simulink model "simulering_ROV_SM_controller"  (R2020a)
settings: Solver=ode45  StartTime=0.0  StopTime=t_sim  RelTol=1e-3
values from neighbouring files (symbols this model uses):
  B = [b11 b12 b13 b14 b15 b16 ... (first row only)    [constants.m]    (also in constants_dp_model.m; constants_model_coriolis.m; constants_process_model.m)
  B_psinv = B'/(B*B')    [constants_dp_model.m]    (also in constants_model_coriolis.m)
  d_11 = 250    [constants.m]    (also in constants_dp_model.m; constants_model_coriolis.m; constants_process_model.m)
  d_22 = 200    [constants.m]    (also in constants_dp_model.m; constants_model_coriolis.m; constants_process_model.m)
  d_33 = 175    [constants.m]    (also in constants_dp_model.m; constants_model_coriolis.m; constants_process_model.m)
  d_44 = 20    [constants.m]    (also in constants_dp_model.m = 15; constants_model_coriolis.m = 15; constants_process_model.m)
  g_z = 9.81    [run_simulation_FL_controller.m]    (also in run_simulation_PID_controller.m = 0.91; run_simulation_SM_controller.m = 0.91; run_simulation_STA_controller.m = 0.91; run_simulation_dp_model.m)
  gamma_r = 0.1    [run_simulation_FL_controller.m]    (also in run_simulation_PID_controller.m; run_simulation_SM_controller.m; run_simulation_STA_controller.m; run_simulation_feedback_linearizing.m)
  gamma_u = 0.1    [run_simulation_FL_controller.m]    (also in run_simulation_PID_controller.m; run_simulation_SM_controller.m; run_simulation_STA_controller.m; run_simulation_feedback_linearizing.m)
  gamma_v = 0.1    [run_simulation_FL_controller.m]    (also in run_simulation_PID_controller.m; run_simulation_SM_controller.m; run_simulation_STA_controller.m; run_simulation_feedback_linearizing.m)
  k_p_psi = wn_psi^2-lambda*k_p_r    [run_simulation_FL_controller.m]    (also in run_simulation_PID_controller.m = wn_psi^2*m_44; run_simulation_dp_model.m = wn_psi^2*m_44; run_simulation_feedback_linearizing.m = tau_r_max/deg2rad(45); run_simulation_feedback_linearizing_second_try.m = wn_psi^2*m_44)
  k_p_u = m_11*pole_u-d_11    [run_simulation_FL_controller.m]    (also in run_simulation_PID_controller.m = 10; run_simulation_dp_model.m = 3; run_simulation_feedback_linearizing.m = tau_u_max/100; run_simulation_feedback_linearizing_second_try.m = 1)
  k_p_v = m_22*pole_v-d_22    [run_simulation_FL_controller.m]    (also in run_simulation_PID_controller.m = 10; run_simulation_dp_model.m = 3; run_simulation_feedback_linearizing.m = tau_v_max/100; run_simulation_feedback_linearizing_second_try.m = 1)
  k_p_z = wn_heave^2*m_33    [run_simulation_PID_controller.m]    (also in tuning_FL_controller.m; tuning_PID_controller.m; tuning_dp_model.m)
  k_s_psi = 50    [run_simulation_SM_controller.m]    (also in tuning_SM_controller.m)
  k_s_u = 500    [run_simulation_SM_controller.m]    (also in tuning_SM_controller.m)
  k_s_v = 400    [run_simulation_SM_controller.m]    (also in tuning_SM_controller.m)
  k_s_z = 10    [run_simulation_SM_controller.m]    (also in tuning_SM_controller.m)
  lambda = d_44    [run_simulation_FL_controller.m]    (also in run_simulation_PID_controller.m = 1; run_simulation_SM_controller.m = 1; run_simulation_STA_controller.m = 1; run_simulation_feedback_linearizing.m = 1)
  lambda_psi = 1    [run_simulation_SM_controller.m]    (also in run_simulation_STA_controller.m = 0.5; tuning_SM_controller.m; tuning_STA_controller.m = 0.5)
  lambda_u = 0.5    [run_simulation_SM_controller.m]    (also in run_simulation_STA_controller.m = 10; tuning_SM_controller.m; tuning_STA_controller.m = 10)
  lambda_v = 0.5    [run_simulation_SM_controller.m]    (also in run_simulation_STA_controller.m = 10; tuning_SM_controller.m; tuning_STA_controller.m = 10)
  lambda_z = 3    [run_simulation_SM_controller.m]    (also in tuning_SM_controller.m)
  m_11 = m_RB11+m_A11    (= 144)    [constants.m]    (also in constants_dp_model.m; constants_model_coriolis.m; constants_process_model.m)
  m_22 = m_RB22+m_A22    (= 162)    [constants.m]    (also in constants_dp_model.m; constants_model_coriolis.m; constants_process_model.m)
  m_44 = m_RB44+m_A44    (= 21)    [constants.m]    (also in constants_dp_model.m = 18.2; constants_model_coriolis.m = 18.2; constants_process_model.m)
  m_A11 = 54    [constants.m]    (also in constants_dp_model.m; constants_model_coriolis.m; constants_process_model.m)
  m_A22 = 72    [constants.m]    (also in constants_dp_model.m; constants_model_coriolis.m; constants_process_model.m)
  m_A33 = 360    [constants.m]    (also in constants_dp_model.m; constants_model_coriolis.m; constants_process_model.m)
  m_A44 = 11    [constants.m]    (also in constants_dp_model.m = 5.2; constants_model_coriolis.m = 5.2; constants_process_model.m)
  m_RB11 = 90    [constants.m]    (also in constants_dp_model.m; constants_model_coriolis.m; constants_process_model.m)
  m_RB22 = 90    [constants.m]    (also in constants_dp_model.m; constants_model_coriolis.m; constants_process_model.m)
  m_RB33 = 90    [constants.m]    (also in constants_dp_model.m; constants_model_coriolis.m; constants_process_model.m)
  m_RB44 = 10    [constants.m]    (also in constants_dp_model.m = 13; constants_model_coriolis.m = 13; constants_process_model.m)
  phi_psi = 0.5    [run_simulation_SM_controller.m]    (also in tuning_SM_controller.m)
  phi_u = 1    [run_simulation_SM_controller.m]    (also in tuning_SM_controller.m)
  phi_v = 1    [run_simulation_SM_controller.m]    (also in tuning_SM_controller.m)
  phi_z = 0.5    [run_simulation_SM_controller.m]    (also in tuning_SM_controller.m)
  psi0 = deg2rad(psi0)    [constants.m]    (also in constants_dp_model.m; constants_model_coriolis.m; constants_process_model.m)
  r0 = 0    [constants.m]    (also in constants_dp_model.m; constants_model_coriolis.m; constants_process_model.m)
  u0 = 0    [constants.m]    (also in constants_dp_model.m; constants_model_coriolis.m; constants_process_model.m)
  v0 = 0    [constants.m]    (also in constants_dp_model.m; constants_model_coriolis.m; constants_process_model.m)
  V_x = 1    [constants.m]    (also in constants_process_model.m; run_simulation_FL_controller.m = 0.25; run_simulation_PID_controller.m = 0.25; run_simulation_dp_model.m = 0.25)
  V_y = 0    [constants.m]    (also in constants_process_model.m; run_simulation_FL_controller.m = -0.6; run_simulation_PID_controller.m = -0.6; run_simulation_dp_model.m = -0.6)
  w0 = 0    [constants.m]    (also in constants_dp_model.m; constants_model_coriolis.m; constants_process_model.m)
  x0 = -2*50    (= -100)    [constants.m]    (also in constants_dp_model.m = 0; constants_model_coriolis.m = 0; constants_process_model.m = 0)
  y0 = 0    [constants.m]    (also in constants_dp_model.m; constants_model_coriolis.m; constants_process_model.m)
  z0 = 0    [constants.m]    (also in constants_dp_model.m; constants_model_coriolis.m; constants_process_model.m)
settings Model: Creator=kenng  LastModifiedBy=kenng

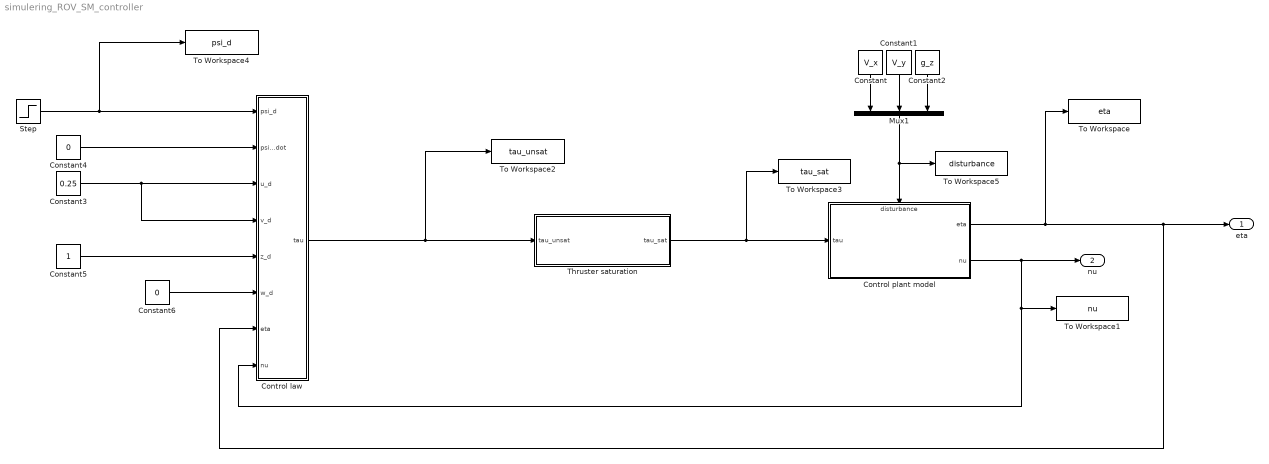
== system simulering_ROV_SM_controller ==
  Constant : Constant  Value=V_x
  Constant1 : Constant  Value=V_y
  Constant2 : Constant  Value=g_z
  Constant3 : Constant  Value=0.25
  Constant4 : Constant  Value=0
  Constant5 : Constant
  Constant6 : Constant  Value=0
  Control law : Subsystem
  Control plant model : Subsystem
      settings: PortSchema="{\"entries\":[{\"content\":{\"sides\":[{\"content\":{\"connectorIds\":[\"In1\"]},\"type\":\"ConnectorPlacement.EquallySpacedRectSide\",\"uuid\":\"e717a587-3200-458e-ba24-dd41565550b9\"},{\"content\":{\"connectorIds\":[\"Out1\",\"Out2\"],\"side\":\"RIGHT\"},\"type\":\"ConnectorPlacement.EquallySpacedRectSide\",\"uuid\":\"302c9cc9-c34e-45c2-bf93-40982187bd66\"},{\"content\":{\"connectorIds\":[\"In2\"],\"side\":\"TOP\"},\"type\":\"ConnectorPlacement.EquallySpacedRectSide\",\"uuid\":\"4b1c13ad-6fa1-447d-8a08-ad292496a8ea\"}]},\"type\":\"ConnectorPlacement.EquallySpacedConnector\",\"uuid\":\"78ff5622-69b9-4402-ac71-5e2cc2861626\"}],\"packageUris\":[\"http://schema.mathworks.com/mf0/Connector/19700101\"],\"version\":\"1.0\"}"
  Mux1 : Mux  Inputs=3
  Step : Step  Time=1000  Before=deg2rad(45)  After=deg2rad(90)  SampleTime=0
  Thruster saturation : Subsystem
  To Workspace : ToWorkspace  VariableName=eta  SaveFormat=Structure With Time  SampleTime=-1
  To Workspace1 : ToWorkspace  VariableName=nu  SaveFormat=Structure With Time  SampleTime=-1
  To Workspace2 : ToWorkspace  VariableName=tau_unsat  SaveFormat=Structure With Time  SampleTime=-1
  To Workspace3 : ToWorkspace  VariableName=tau_sat  SaveFormat=Structure With Time  SampleTime=-1
  To Workspace4 : ToWorkspace  VariableName=psi_d  SaveFormat=Structure With Time  SampleTime=-1
  To Workspace5 : ToWorkspace  VariableName=disturbance  SaveFormat=Structure With Time  SampleTime=-1
  eta : Outport
  nu : Outport  Port=2
  wires:
  Control plant model/1(eta) -> To Workspace/1, Control law/7(eta), eta/1
  Control plant model/2(nu) -> nu/1, To Workspace1/1, Control law/8(nu)
  Mux1/1 -> To Workspace5/1, Control plant model/2(disturbance)
  Control law/1(tau) -> Thruster saturation/1(tau_unsat), To Workspace2/1
  Step/1 -> To Workspace4/1, Control law/1(psi_d)
  Constant3/1 -> Control law/4(v_d), Control law/3(u_d)
  Constant/1 -> Mux1/1
  Constant1/1 -> Mux1/2
  Constant2/1 -> Mux1/3
  Constant5/1 -> Control law/5(z_d)
  Thruster saturation/1(tau_sat) -> To Workspace3/1, Control plant model/1(tau)
  Constant4/1 -> Control law/2(psi_d_dot)
  Constant6/1 -> Control law/6(w_d)

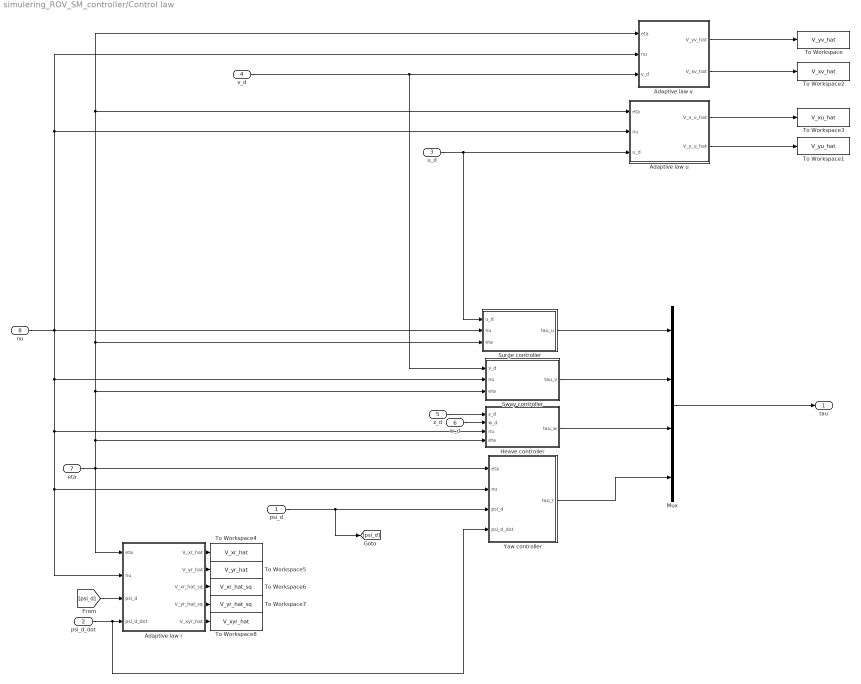
== system simulering_ROV_SM_controller/Control law ==
  psi_d : Inport
  psi_d_dot : Inport  Port=2
  u_d : Inport  Port=3
  v_d : Inport  Port=4
  z_d : Inport  Port=5
  w_d : Inport  Port=6
  eta : Inport  Port=7
  nu : Inport  Port=8
  Adaptive law r : Subsystem
  Adaptive law u : Subsystem
  Adaptive law v : Subsystem
  Heave controller : Subsystem
  Mux : Mux
  Surge controller : Subsystem
  Sway controller : Subsystem
  To Workspace : ToWorkspace  VariableName=V_yv_hat  SaveFormat=Structure With Time  SampleTime=-1
  To Workspace1 : ToWorkspace  VariableName=V_yu_hat  SaveFormat=Structure With Time  SampleTime=-1
  To Workspace2 : ToWorkspace  VariableName=V_xv_hat  SaveFormat=Structure With Time  SampleTime=-1
  To Workspace3 : ToWorkspace  VariableName=V_xu_hat  SaveFormat=Structure With Time  SampleTime=-1
  To Workspace4 : ToWorkspace  VariableName=V_xr_hat  SaveFormat=Structure With Time  SampleTime=-1
  To Workspace5 : ToWorkspace  VariableName=V_yr_hat  SaveFormat=Structure With Time  SampleTime=-1
  To Workspace6 : ToWorkspace  VariableName=V_xr_hat_sq  SaveFormat=Structure With Time  SampleTime=-1
  To Workspace7 : ToWorkspace  VariableName=V_yr_hat_sq  SaveFormat=Structure With Time  SampleTime=-1
  To Workspace8 : ToWorkspace  VariableName=V_xyr_hat  SaveFormat=Structure With Time  SampleTime=-1
  Yaw controller : Subsystem
  tau : Outport
  wires:
  Heave controller/1(tau_w) -> Mux/3
  Mux/1 -> tau/1
  u_d/1 -> Surge controller/1(u_d), Adaptive law u/3(u_d)
  v_d/1 -> Adaptive law v/3(v_d), Sway controller/1(v_d)
  z_d/1 -> Heave controller/1(z_d)
  Adaptive law u/2(V_y_u_hat) -> To Workspace1/1
  Adaptive law u/1(V_x_u_hat) -> To Workspace3/1
  Adaptive law v/1(V_yv_hat) -> To Workspace/1
  Adaptive law v/2(V_xv_hat) -> To Workspace2/1
  Adaptive law r/1(V_xr_hat) -> To Workspace4/1
  Adaptive law r/2(V_yr_hat) -> To Workspace5/1
  Adaptive law r/3(V_xr_hat_sq) -> To Workspace6/1
  Adaptive law r/4(V_yr_hat_sq) -> To Workspace7/1
  Adaptive law r/5(V_xyr_hat) -> To Workspace8/1
  [psi_d] -> Adaptive law r/3(psi_d)
  psi_d_dot/1 -> Yaw controller/4(psi_d_dot), Adaptive law r/4(psi_d_dot)
  eta/1 -> Adaptive law u/1(eta), Adaptive law v/1(eta), Surge controller/3(eta), Sway controller/3(eta), Heave controller/4(eta), Adaptive law r/1(eta), Yaw controller/1(eta)
  nu/1 -> Adaptive law r/2(nu), Yaw controller/2(nu), Heave controller/3(nu), Sway controller/2(nu), Adaptive law u/2(nu), Adaptive law v/2(nu), Surge controller/2(nu)
  psi_d/1 -> Yaw controller/3(psi_d), [psi_d]
  Yaw controller/1(tau_r) -> Mux/4
  Surge controller/1(tau_u) -> Mux/1
  Sway controller/1(tau_v) -> Mux/2
  w_d/1 -> Heave controller/2(w_d)

== system simulering_ROV_SM_controller/Control plant model ==
  note: tau: 4x1 vector = [surge sway heave yaw]^T
  note: Disturbance: 3x1 vector = [Vx Vy gz]^t
  tau : Inport
  disturbance : Inport  Port=2
  Demux : Demux
  Kinematics : Subsystem
  Kinetics : Subsystem
  Terminator : Terminator
  Terminator1 : Terminator
  Terminator2 : Terminator
  eta : Outport
  nu : Outport  Port=2
  wires:
  tau/1 -> Kinetics/2(tau)
  Kinetics/1(nu) -> nu/1, Kinematics/1(nu)
  Demux/4 -> Kinetics/3(psi)
  Demux/2 -> Terminator1/1
  Kinematics/1(eta) -> eta/1, Demux/1
  Demux/1 -> Terminator/1
  Demux/3 -> Terminator2/1
  disturbance/1 -> Kinetics/1(disturbance)

== system simulering_ROV_SM_controller/Thruster saturation ==
  tau_unsat : Inport
  Constant : Constant  Value=B_psinv
  Constant1 : Constant  Value=B
  Demux : Demux  Outputs=6
  Matrix Multiply : Product  Multiplication=Matrix(*)
  Matrix Multiply1 : Product  Multiplication=Matrix(*)
  Mux : Mux  Inputs=6
  Saturation{,1..5} (6 alike) : Saturate  UpperLimit=120  LowerLimit=-120
  tau_sat : Outport
  wires:
  tau_unsat/1 -> Matrix Multiply/2
  Constant/1 -> Matrix Multiply/1
  Matrix Multiply/1 -> Demux/1
  Demux/2 -> Saturation1/1
  Demux/1 -> Saturation/1
  Demux/3 -> Saturation2/1
  Demux/4 -> Saturation3/1
  Demux/5 -> Saturation4/1
  Demux/6 -> Saturation5/1
  Saturation/1 -> Mux/1
  Saturation1/1 -> Mux/2
  Saturation2/1 -> Mux/3
  Saturation3/1 -> Mux/4
  Saturation4/1 -> Mux/5
  Saturation5/1 -> Mux/6
  Mux/1 -> Matrix Multiply1/2
  Constant1/1 -> Matrix Multiply1/1
  Matrix Multiply1/1 -> tau_sat/1

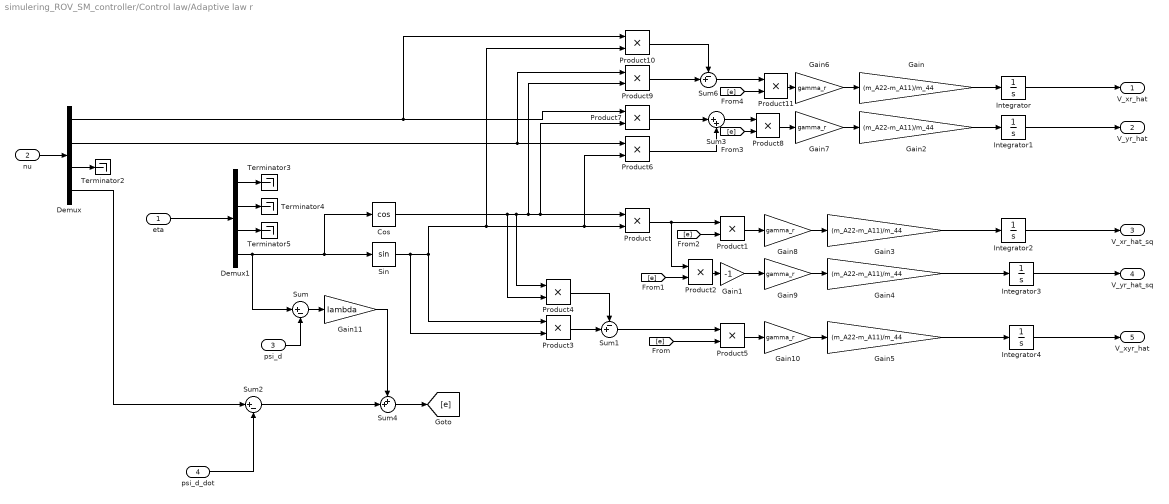
== system simulering_ROV_SM_controller/Control law/Adaptive law r ==
  eta : Inport
  nu : Inport  Port=2
  psi_d : Inport  Port=3
  psi_d_dot : Inport  Port=4
  Cos : Trigonometry  Operator=cos
  Demux : Demux
  Demux1 : Demux
  Gain{,2..5} (5 alike) : Gain  Gain=(m_A22-m_A11)/m_44
  Gain1 : Gain  Gain=-1
  Gain{6..10} (5 alike) : Gain  Gain=gamma_r
  Gain11 : Gain  Gain=lambda
  Integrator{,1..4} (5 alike) : Integrator
  Product{,1..11} (12 alike) : Product
  Sin : Trigonometry
  Sum : Sum  Inputs=|+-
  Sum1 : Sum  Inputs=-+|
  Sum2 : Sum  Inputs=|+-
  Sum3 : Sum  Inputs=|++
  Sum4 : Sum  Inputs=++|
  Sum6 : Sum  Inputs=-+|
  Terminator{2..5} (4 alike) : Terminator
  V_xr_hat : Outport
  V_yr_hat : Outport  Port=2
  V_xr_hat_sq : Outport  Port=3
  V_yr_hat_sq : Outport  Port=4
  V_xyr_hat : Outport  Port=5
  wires:
  [e] -> Product11/2
  [e] -> Product8/2
  nu/1 -> Demux/1
  Demux/1 -> Product10/1, Product7/1
  Demux/2 -> Product9/1, Product6/1
  Demux/3 -> Terminator2/1
  Demux1/2 -> Terminator4/1
  eta/1 -> Demux1/1
  Demux1/1 -> Terminator3/1
  Demux1/3 -> Terminator5/1
  Demux1/4 -> Cos/1, Sin/1, Sum/1
  Demux/4 -> Sum2/1
  Sin/1 -> Product3/2, Product3/1, Product10/2, Product6/2, Product/2
  Cos/1 -> Product4/2, Product4/1, Product9/2, Product7/2, Product/1
  [e] -> Product1/2
  Product1/1 -> Gain8/1
  Product2/1 -> Gain1/1
  [e] -> Product2/2
  Product/1 -> Product2/1, Product1/1
  Product3/1 -> Sum1/2
  Product4/1 -> Sum1/1
  Sum1/1 -> Product5/1
  [e] -> Product5/2
  Product7/1 -> Sum3/1
  Product6/1 -> Sum3/2
  Sum3/1 -> Product8/1
  Product9/1 -> Sum6/2
  Product10/1 -> Sum6/1
  Sum6/1 -> Product11/1
  Gain1/1 -> Gain9/1
  Product11/1 -> Gain6/1
  Product8/1 -> Gain7/1
  Product5/1 -> Gain10/1
  Gain/1 -> Integrator/1
  Gain2/1 -> Integrator1/1
  Gain3/1 -> Integrator2/1
  Gain4/1 -> Integrator3/1
  Gain5/1 -> Integrator4/1
  Integrator4/1 -> V_xyr_hat/1
  Integrator3/1 -> V_yr_hat_sq/1
  Integrator2/1 -> V_xr_hat_sq/1
  Integrator1/1 -> V_yr_hat/1
  Integrator/1 -> V_xr_hat/1
  Gain6/1 -> Gain/1
  Gain7/1 -> Gain2/1
  Gain8/1 -> Gain3/1
  Gain9/1 -> Gain4/1
  Gain10/1 -> Gain5/1
  psi_d_dot/1 -> Sum2/2
  psi_d/1 -> Sum/2
  Sum/1 -> Gain11/1
  Sum2/1 -> Sum4/2
  Gain11/1 -> Sum4/1
  Sum4/1 -> [e]

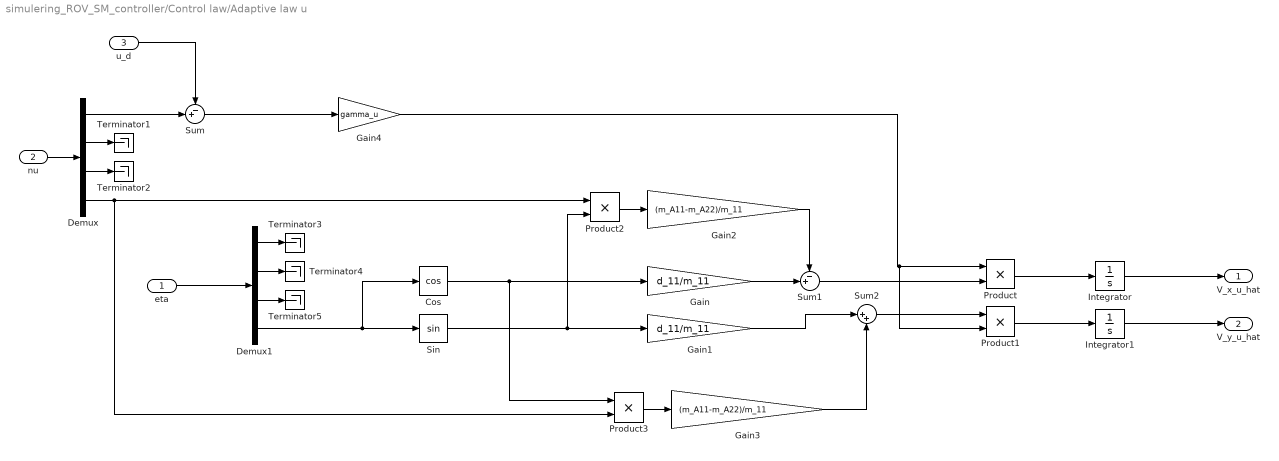
== system simulering_ROV_SM_controller/Control law/Adaptive law u ==
  eta : Inport
  nu : Inport  Port=2
  u_d : Inport  Port=3
  Cos : Trigonometry  Operator=cos
  Demux : Demux
  Demux1 : Demux
  Gain : Gain  Gain=d_11/m_11
  Gain1 : Gain  Gain=d_11/m_11
  Gain2 : Gain  Gain=(m_A11-m_A22)/m_11
  Gain3 : Gain  Gain=(m_A11-m_A22)/m_11
  Gain4 : Gain  Gain=gamma_u
  Integrator : Integrator
  Integrator1 : Integrator
  Product{,1..3} (4 alike) : Product
  Sin : Trigonometry
  Sum : Sum  Inputs=-+|
  Sum1 : Sum  Inputs=-+|
  Sum2 : Sum  Inputs=|++
  Terminator{1..5} (5 alike) : Terminator
  V_x_u_hat : Outport
  V_y_u_hat : Outport  Port=2
  wires:
  Sin/1 -> Product2/2, Gain1/1
  Product/1 -> Integrator/1
  Product1/1 -> Integrator1/1
  Gain4/1 -> Product1/2, Product/1
  Integrator/1 -> V_x_u_hat/1
  Gain/1 -> Sum1/2
  Sum1/1 -> Product/2
  Gain2/1 -> Sum1/1
  nu/1 -> Demux/1
  Product2/1 -> Gain2/1
  Sum2/1 -> Product1/1
  Gain1/1 -> Sum2/1
  Product3/1 -> Gain3/1
  Cos/1 -> Product3/1, Gain/1
  Gain3/1 -> Sum2/2
  Demux/4 -> Product2/1, Product3/2
  Demux/1 -> Sum/2
  Demux/2 -> Terminator1/1
  Demux/3 -> Terminator2/1
  Demux1/2 -> Terminator4/1
  eta/1 -> Demux1/1
  Demux1/1 -> Terminator3/1
  Demux1/3 -> Terminator5/1
  Demux1/4 -> Cos/1, Sin/1
  u_d/1 -> Sum/1
  Sum/1 -> Gain4/1
  Integrator1/1 -> V_y_u_hat/1

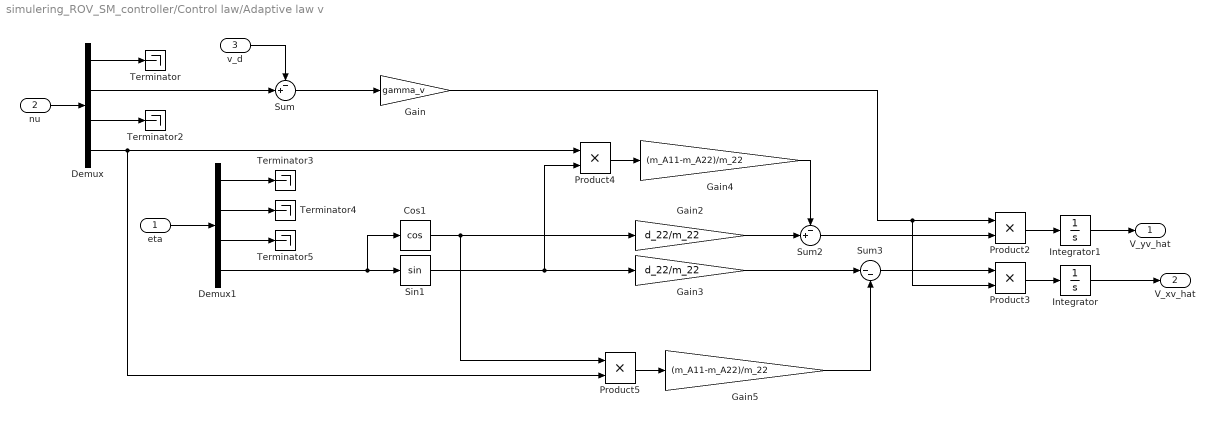
== system simulering_ROV_SM_controller/Control law/Adaptive law v ==
  eta : Inport
  nu : Inport  Port=2
  v_d : Inport  Port=3
  Cos1 : Trigonometry  Operator=cos
  Demux : Demux
  Demux1 : Demux
  Gain : Gain  Gain=gamma_v
  Gain2 : Gain  Gain=d_22/m_22
  Gain3 : Gain  Gain=d_22/m_22
  Gain4 : Gain  Gain=(m_A11-m_A22)/m_22
  Gain5 : Gain  Gain=(m_A11-m_A22)/m_22
  Integrator : Integrator
  Integrator1 : Integrator
  Product{2..5} (4 alike) : Product
  Sin1 : Trigonometry
  Sum : Sum  Inputs=-+|
  Sum2 : Sum  Inputs=-+|
  Sum3 : Sum  Inputs=|--
  Terminator{,2..5} (5 alike) : Terminator
  V_yv_hat : Outport
  V_xv_hat : Outport  Port=2
  wires:
  Gain4/1 -> Sum2/1
  Product5/1 -> Gain5/1
  Gain2/1 -> Sum2/2
  Demux/3 -> Terminator2/1
  Product4/1 -> Gain4/1
  nu/1 -> Demux/1
  Gain5/1 -> Sum3/2
  Sum2/1 -> Product2/2
  Integrator1/1 -> V_yv_hat/1
  Gain/1 -> Product3/2, Product2/1
  Product2/1 -> Integrator1/1
  Sum3/1 -> Product3/1
  Demux/2 -> Sum/2
  Demux/1 -> Terminator/1
  Gain3/1 -> Sum3/1
  Demux/4 -> Product4/1, Product5/2
  Cos1/1 -> Product5/1, Gain2/1
  Sin1/1 -> Product4/2, Gain3/1
  Demux1/1 -> Terminator3/1
  Demux1/2 -> Terminator4/1
  eta/1 -> Demux1/1
  Demux1/3 -> Terminator5/1
  Demux1/4 -> Cos1/1, Sin1/1
  Product3/1 -> Integrator/1
  Integrator/1 -> V_xv_hat/1
  v_d/1 -> Sum/1
  Sum/1 -> Gain/1

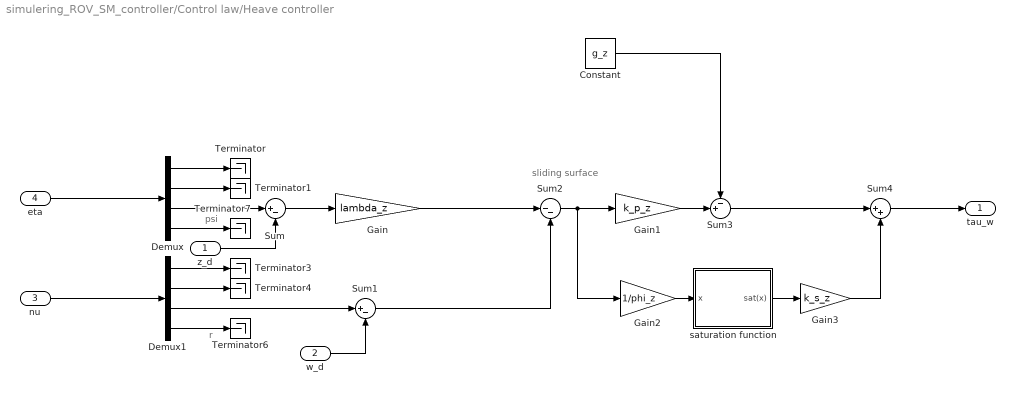
== system simulering_ROV_SM_controller/Control law/Heave controller ==
  note: sliding surface
  note: r
  note: psi
  z_d : Inport
  w_d : Inport  Port=2
  nu : Inport  Port=3
  eta : Inport  Port=4
  Constant : Constant  Value=g_z
  Demux : Demux
  Demux1 : Demux
  Gain : Gain  Gain=lambda_z
  Gain1 : Gain  Gain=k_p_z
  Gain2 : Gain  Gain=1/phi_z
  Gain3 : Gain  Gain=k_s_z
  Sum : Sum  Inputs=|+-
  Sum1 : Sum  Inputs=|+-
  Sum2 : Sum  Inputs=|--
  Sum3 : Sum  Inputs=-+|
  Sum4 : Sum  Inputs=|++
  Terminator{,1,3..4,6..7} (6 alike) : Terminator
  saturation function : Subsystem
  tau_w : Outport
  wires:
  Demux1/2 -> Terminator4/1
  Demux/1 -> Terminator/1
  eta/1 -> Demux/1
  Demux/2 -> Terminator1/1
  Demux1/1 -> Terminator3/1
  Demux/3 -> Sum/1
  nu/1 -> Demux1/1
  Demux1/4 -> Terminator6/1
  Demux/4 -> Terminator7/1
  z_d/1 -> Sum/2
  Sum/1 -> Gain/1
  Demux1/3 -> Sum1/1
  w_d/1 -> Sum1/2
  Gain/1 -> Sum2/1
  Sum1/1 -> Sum2/2
  Sum2/1 -> Gain2/1, Gain1/1
  Constant/1 -> Sum3/1
  Gain1/1 -> Sum3/2
  Gain2/1 -> saturation function/1(x)
  Sum3/1 -> Sum4/1
  saturation function/1(sat(x)) -> Gain3/1
  Gain3/1 -> Sum4/2
  Sum4/1 -> tau_w/1

== system simulering_ROV_SM_controller/Control law/Surge controller ==
  note: sliding surface
  note: r
  note: psi
  u_d : Inport
  nu : Inport  Port=2
  eta : Inport  Port=3
  Demux : Demux
  Demux1 : Demux
  Gain : Gain  Gain=lambda_u
  Gain1 : Gain  Gain=k_p_u
  Gain2 : Gain  Gain=1/phi_u
  Gain3 : Gain  Gain=k_s_u
  Integrator : Integrator
  Sum : Sum  Inputs=|+-
  Sum1 : Sum  Inputs=|--
  Sum2 : Sum  Inputs=|++
  Terminator{,1..2,4..7} (7 alike) : Terminator
  saturation function : Subsystem
  tau_u : Outport
  wires:
  Demux1/2 -> Terminator4/1
  eta/1 -> Demux/1
  Demux/2 -> Terminator1/1
  Demux1/1 -> Sum/1
  nu/1 -> Demux1/1
  Demux1/4 -> Terminator6/1
  Demux/4 -> Terminator7/1
  u_d/1 -> Sum/2
  Demux1/3 -> Terminator2/1
  Demux/3 -> Terminator/1
  Demux/1 -> Terminator5/1
  Sum/1 -> Integrator/1, Sum1/2
  Integrator/1 -> Gain/1
  Gain/1 -> Sum1/1
  Sum1/1 -> Gain2/1, Gain1/1
  Gain2/1 -> saturation function/1(x)
  saturation function/1(sat(x)) -> Gain3/1
  Gain1/1 -> Sum2/1
  Gain3/1 -> Sum2/2
  Sum2/1 -> tau_u/1

== system simulering_ROV_SM_controller/Control law/Sway controller ==
  note: sliding surface
  note: r
  note: psi
  v_d : Inport
  nu : Inport  Port=2
  eta : Inport  Port=3
  Demux : Demux
  Demux1 : Demux
  Gain : Gain  Gain=k_p_v
  Gain1 : Gain  Gain=lambda_v
  Gain2 : Gain  Gain=1/phi_v
  Gain3 : Gain  Gain=k_s_v
  Integrator : Integrator
  Sum : Sum  Inputs=|+-
  Sum1 : Sum  Inputs=|--
  Sum2 : Sum  Inputs=|++
  Terminator{,1..3,5..7} (7 alike) : Terminator
  saturation function : Subsystem
  tau_v : Outport
  wires:
  Demux1/2 -> Sum/1
  Demux/1 -> Terminator/1
  eta/1 -> Demux/1
  Demux1/1 -> Terminator3/1
  nu/1 -> Demux1/1
  Demux1/4 -> Terminator6/1
  Demux/4 -> Terminator7/1
  v_d/1 -> Sum/2
  Gain/1 -> Sum2/1
  Demux1/3 -> Terminator2/1
  Demux/3 -> Terminator1/1
  Demux/2 -> Terminator5/1
  Sum/1 -> Sum1/2, Integrator/1
  Integrator/1 -> Gain1/1
  Sum1/1 -> Gain2/1, Gain/1
  Gain2/1 -> saturation function/1(x)
  saturation function/1(sat(x)) -> Gain3/1
  Gain3/1 -> Sum2/2
  Sum2/1 -> tau_v/1
  Gain1/1 -> Sum1/1

== system simulering_ROV_SM_controller/Control law/Yaw controller ==
  note: sliding surface
  note: r
  note: psi
  eta : Inport
  nu : Inport  Port=2
  psi_d : Inport  Port=3
  psi_d_dot : Inport  Port=4
  Demux : Demux
  Demux1 : Demux
  Gain : Gain  Gain=lambda_psi
  Gain1 : Gain  Gain=1/phi_psi
  Gain2 : Gain  Gain=k_p_psi
  Gain3 : Gain  Gain=k_s_psi
  SSA : MATLAB Function  TreatAsAtomicUnit=on
  Sum : Sum  Inputs=|+-
  Sum1 : Sum  Inputs=|+-
  Sum2 : Sum  Inputs=|--
  Sum4 : Sum  Inputs=|++
  Terminator{,1..5} (6 alike) : Terminator
  saturation function : Subsystem
  tau_r : Outport
  wires:
  Demux/2 -> Terminator1/1
  Demux/1 -> Terminator/1
  Demux1/1 -> Terminator3/1
  Demux1/3 -> Terminator2/1
  Demux1/2 -> Terminator4/1
  eta/1 -> Demux/1
  nu/1 -> Demux1/1
  Demux/3 -> Terminator5/1
  Gain2/1 -> Sum4/1
  Sum4/1 -> tau_r/1
  psi_d/1 -> Sum/2
  Demux/4 -> Sum/1
  Demux1/4 -> Sum1/1
  psi_d_dot/1 -> Sum1/2
  Sum/1 -> SSA/1(u)
  Gain/1 -> Sum2/1
  Sum1/1 -> Sum2/2
  Sum2/1 -> Gain1/1, Gain2/1
  Gain1/1 -> saturation function/1(x)
  saturation function/1(sat(x)) -> Gain3/1
  Gain3/1 -> Sum4/2
  SSA/1(y) -> Gain/1

== system simulering_ROV_SM_controller/Control plant model/Kinematics ==
  nu : Inport
  Cos : Trigonometry  Operator=cos
  Demux : Demux
  Integrator : Integrator  InitialCondition=psi0
  Integrator1 : Integrator  InitialCondition=z0
  Integrator2 : Integrator  InitialCondition=x0
  Integrator3 : Integrator  InitialCondition=y0
  Mux : Mux
  Product{,1..3} (4 alike) : Product
  Sin : Trigonometry
  Sum : Sum  Inputs=|++
  Sum1 : Sum  Inputs=|+-
  eta : Outport
  wires:
  Sin/1 -> [sinpsi]
  Demux/3 -> Integrator1/1
  Demux/1 -> Product1/1, Product/1
  Demux/2 -> Product3/1, Product2/1
  [sinpsi] -> Product3/2
  [psi] -> Sin/1, Cos/1
  [cospsi] -> Product2/2
  Cos/1 -> [cospsi]
  Product1/1 -> Sum/1
  Integrator/1 -> Mux/4, [psi]
  [sinpsi] -> Product1/2
  Product/1 -> Sum1/1
  Sum1/1 -> Integrator2/1
  Demux/4 -> Integrator/1
  Sum/1 -> Integrator3/1
  [cospsi] -> Product/2
  nu/1 -> Demux/1
  Product2/1 -> Sum/2
  Product3/1 -> Sum1/2
  Integrator3/1 -> Mux/2
  Integrator1/1 -> Mux/3
  Integrator2/1 -> Mux/1
  Mux/1 -> eta/1

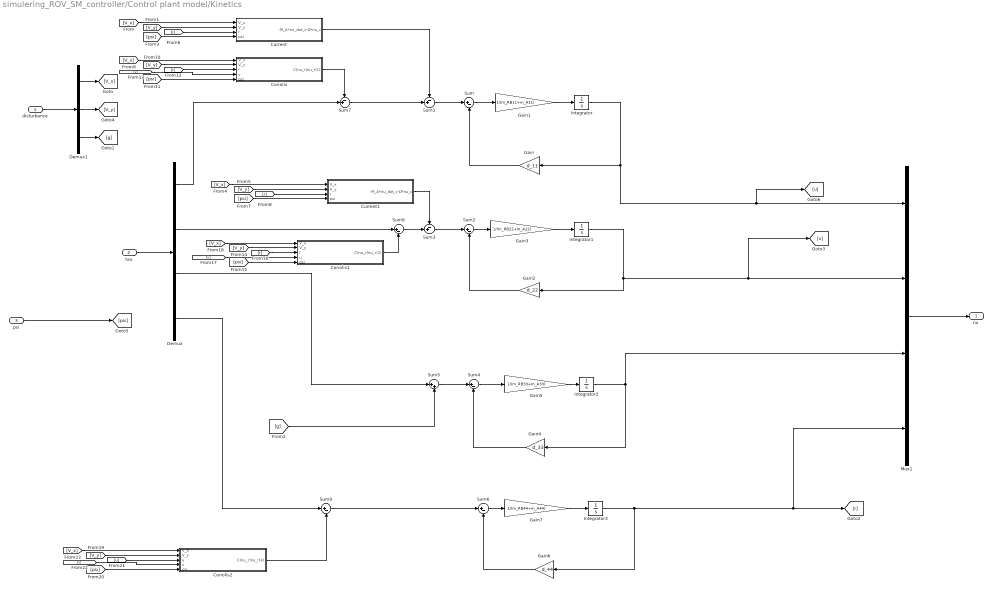
== system simulering_ROV_SM_controller/Control plant model/Kinetics ==
  disturbance : Inport
  tau : Inport  Port=2
  psi : Inport  Port=3
  Coriolis : Subsystem
  Coriolis1 : Subsystem
  Coriolis2 : Subsystem
  Current : Subsystem
  Current1 : Subsystem
  Demux : Demux
  Demux1 : Demux  Outputs=3
  Gain : Gain  Gain=d_11
  Gain1 : Gain  Gain=1/(m_RB11+m_A11)
  Gain2 : Gain  Gain=d_22
  Gain3 : Gain  Gain=1/(m_RB22+m_A22)
  Gain4 : Gain  Gain=d_33
  Gain5 : Gain  Gain=1/(m_RB33+m_A33)
  Gain6 : Gain  Gain=d_44
  Gain7 : Gain  Gain=1/(m_RB44+m_A44)
  Integrator : Integrator  InitialCondition=u0
  Integrator1 : Integrator  InitialCondition=v0
  Integrator2 : Integrator  InitialCondition=w0
  Integrator3 : Integrator  InitialCondition=r0
  Mux1 : Mux
  Sum{,2,4,6,8..9} (6 alike) : Sum  Inputs=|+-
  Sum1 : Sum  Inputs=-+|
  Sum3 : Sum  Inputs=-+|
  Sum5 : Sum  Inputs=|++
  Sum7 : Sum  Inputs=-+|
  nu : Outport
  wires:
  Demux1/1 -> [V_x]
  Gain1/1 -> Integrator/1
  Sum/1 -> Gain1/1
  tau/1 -> Demux/1
  Integrator1/1 -> Gain2/1, [v], Mux1/2
  Gain3/1 -> Integrator1/1
  Mux1/1 -> nu/1
  Integrator/1 -> [u], Mux1/1, Gain/1
  Integrator2/1 -> Gain4/1, Mux1/3
  Gain5/1 -> Integrator2/1
  Demux1/3 -> [g]
  Sum3/1 -> Sum2/1
  Sum4/1 -> Gain5/1
  Gain2/1 -> Sum2/2
  Sum2/1 -> Gain3/1
  Gain/1 -> Sum/2
  Gain4/1 -> Sum4/2
  Sum1/1 -> Sum/1
  Gain6/1 -> Sum6/2
  Demux1/2 -> [V_y]
  [r] -> Current/3(r)
  Integrator3/1 -> [r], Mux1/4, Gain6/1
  disturbance/1 -> Demux1/1
  Sum6/1 -> Gain7/1
  Gain7/1 -> Integrator3/1
  psi/1 -> [psi]
  Current/1(-M_A*nu_dot_c-D*nu_c) -> Sum1/1
  [V_y] -> Current/2(V_y)
  [V_x] -> Current/1(V_x)
  [psi] -> Current/4(psi)
  [r] -> Current1/3(r)
  [psi] -> Current1/4(psi)
  [V_x] -> Current1/1(V_x)
  [V_y] -> Current1/2(V_y)
  Current1/1(-M_A*nu_dot_c-D*nu_c) -> Sum3/1
  [g] -> Sum5/2
  Demux/3 -> Sum5/1
  Sum5/1 -> Sum4/1
  Coriolis/1(C(nu_r)nu_r(1)) -> Sum7/1
  Demux/1 -> Sum7/2
  Sum7/1 -> Sum1/2
  [V_x] -> Coriolis/1(V_x)
  [psi] -> Coriolis/5(psi)
  [r] -> Coriolis/3(r)
  [V_y] -> Coriolis/2(V_y)
  [v] -> Coriolis/4(v)
  [u] -> Coriolis1/4(u)
  Coriolis1/1(C(nu_r)nu_r(2)) -> Sum8/2
  [V_y] -> Coriolis1/2(V_y)
  [psi] -> Coriolis1/5(psi)
  [V_x] -> Coriolis1/1(V_x)
  [r] -> Coriolis1/3(r)
  Sum8/1 -> Sum3/2
  Demux/2 -> Sum8/1
  [v] -> Coriolis2/4(v)
  Coriolis2/1(C(nu_r)nu_r(4)) -> Sum9/2
  [V_y] -> Coriolis2/2(V_y)
  [psi] -> Coriolis2/5(psi)
  [V_x] -> Coriolis2/1(V_x)
  [u] -> Coriolis2/3(u)
  Sum9/1 -> Sum6/1
  Demux/4 -> Sum9/1

== system simulering_ROV_SM_controller/Control law/Heave controller/saturation function ==
  x : Inport
  Abs : Abs
  Sign : Signum
  Switch : Switch  Criteria=u2 > Threshold  Threshold=1
  sat(x) : Outport
  wires:
  x/1 -> Sign/1, Abs/1, Switch/3
  Abs/1 -> Switch/2
  Sign/1 -> Switch/1
  Switch/1 -> sat(x)/1

== system simulering_ROV_SM_controller/Control law/Surge controller/saturation function ==
  x : Inport
  Abs : Abs
  Sign : Signum
  Switch : Switch  Criteria=u2 > Threshold  Threshold=1
  sat(x) : Outport
  wires:
  x/1 -> Sign/1, Abs/1, Switch/3
  Abs/1 -> Switch/2
  Sign/1 -> Switch/1
  Switch/1 -> sat(x)/1

== system simulering_ROV_SM_controller/Control law/Sway controller/saturation function ==
  x : Inport
  Abs : Abs
  Sign : Signum
  Switch : Switch  Criteria=u2 > Threshold  Threshold=1
  sat(x) : Outport
  wires:
  x/1 -> Sign/1, Abs/1, Switch/3
  Abs/1 -> Switch/2
  Sign/1 -> Switch/1
  Switch/1 -> sat(x)/1

== system simulering_ROV_SM_controller/Control law/Yaw controller/saturation function ==
  x : Inport
  Abs : Abs
  Sign : Signum
  Switch : Switch  Criteria=u2 > Threshold  Threshold=1
  sat(x) : Outport
  wires:
  x/1 -> Sign/1, Abs/1, Switch/3
  Abs/1 -> Switch/2
  Sign/1 -> Switch/1
  Switch/1 -> sat(x)/1

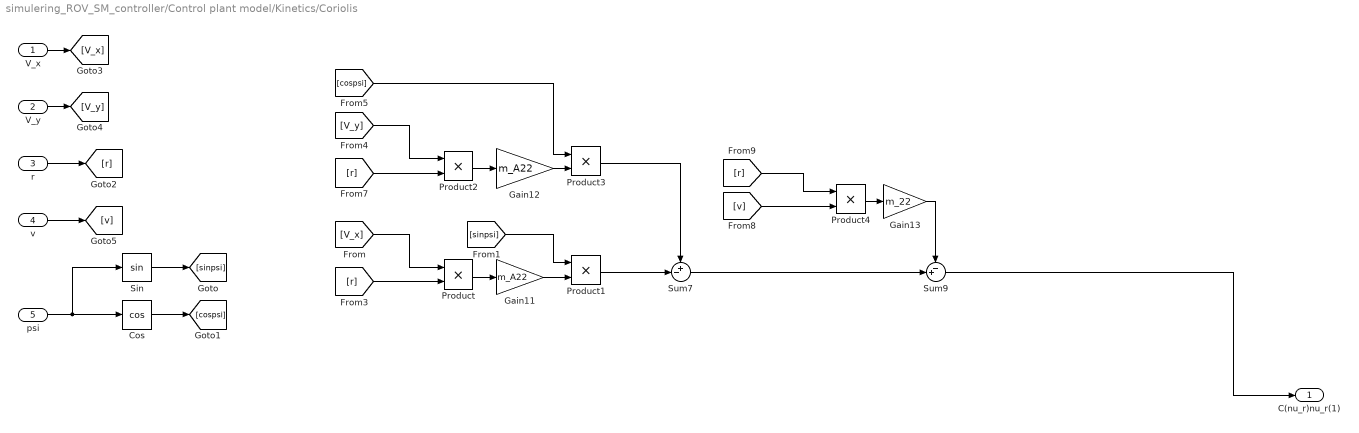
== system simulering_ROV_SM_controller/Control plant model/Kinetics/Coriolis ==
  V_x : Inport
  V_y : Inport  Port=2
  r : Inport  Port=3
  v : Inport  Port=4
  psi : Inport  Port=5
  Cos : Trigonometry  Operator=cos
  Gain11 : Gain  Gain=m_A22
  Gain12 : Gain  Gain=m_A22
  Gain13 : Gain  Gain=m_22
  Product{,1..4} (5 alike) : Product
  Sin : Trigonometry
  Sum7 : Sum  Inputs=+-|
  Sum9 : Sum  Inputs=-+|
  C(nu_r)nu_r(1) : Outport
  wires:
  Gain11/1 -> Product1/2
  Product2/1 -> Gain12/1
  [cospsi] -> Product3/1
  [r] -> Product2/2
  [v] -> Product4/2
  Product4/1 -> Gain13/1
  [V_x] -> Product/1
  Product3/1 -> Sum7/1
  Gain12/1 -> Product3/2
  Product/1 -> Gain11/1
  [V_y] -> Product2/1
  [r] -> Product/2
  Product1/1 -> Sum7/2
  [sinpsi] -> Product1/1
  Sum7/1 -> Sum9/2
  [r] -> Product4/1
  Sum9/1 -> C(nu_r)nu_r(1)/1
  psi/1 -> Sin/1, Cos/1
  Sin/1 -> [sinpsi]
  Cos/1 -> [cospsi]
  r/1 -> [r]
  V_x/1 -> [V_x]
  V_y/1 -> [V_y]
  v/1 -> [v]
  Gain13/1 -> Sum9/1

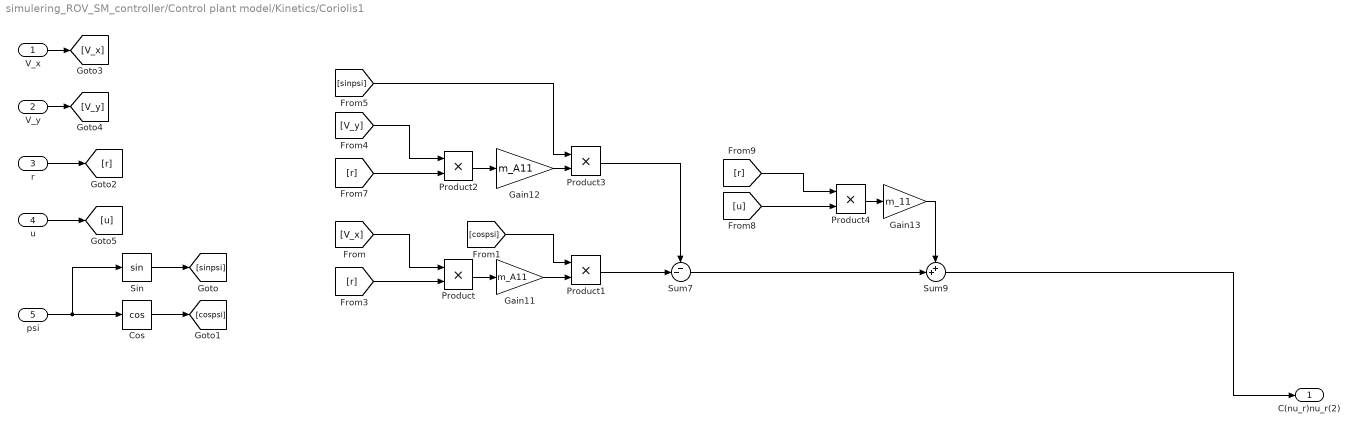
== system simulering_ROV_SM_controller/Control plant model/Kinetics/Coriolis1 ==
  V_x : Inport
  V_y : Inport  Port=2
  r : Inport  Port=3
  u : Inport  Port=4
  psi : Inport  Port=5
  Cos : Trigonometry  Operator=cos
  Gain11 : Gain  Gain=m_A11
  Gain12 : Gain  Gain=m_A11
  Gain13 : Gain  Gain=m_11
  Product{,1..4} (5 alike) : Product
  Sin : Trigonometry
  Sum7 : Sum  Inputs=--|
  Sum9 : Sum  Inputs=++|
  C(nu_r)nu_r(2) : Outport
  wires:
  Gain11/1 -> Product1/2
  Product2/1 -> Gain12/1
  [sinpsi] -> Product3/1
  [r] -> Product2/2
  [u] -> Product4/2
  Product4/1 -> Gain13/1
  [V_x] -> Product/1
  Product3/1 -> Sum7/1
  Gain12/1 -> Product3/2
  Product/1 -> Gain11/1
  [V_y] -> Product2/1
  [r] -> Product/2
  Product1/1 -> Sum7/2
  [cospsi] -> Product1/1
  Sum7/1 -> Sum9/2
  [r] -> Product4/1
  Sum9/1 -> C(nu_r)nu_r(2)/1
  psi/1 -> Sin/1, Cos/1
  Sin/1 -> [sinpsi]
  Cos/1 -> [cospsi]
  r/1 -> [r]
  V_x/1 -> [V_x]
  V_y/1 -> [V_y]
  u/1 -> [u]
  Gain13/1 -> Sum9/1

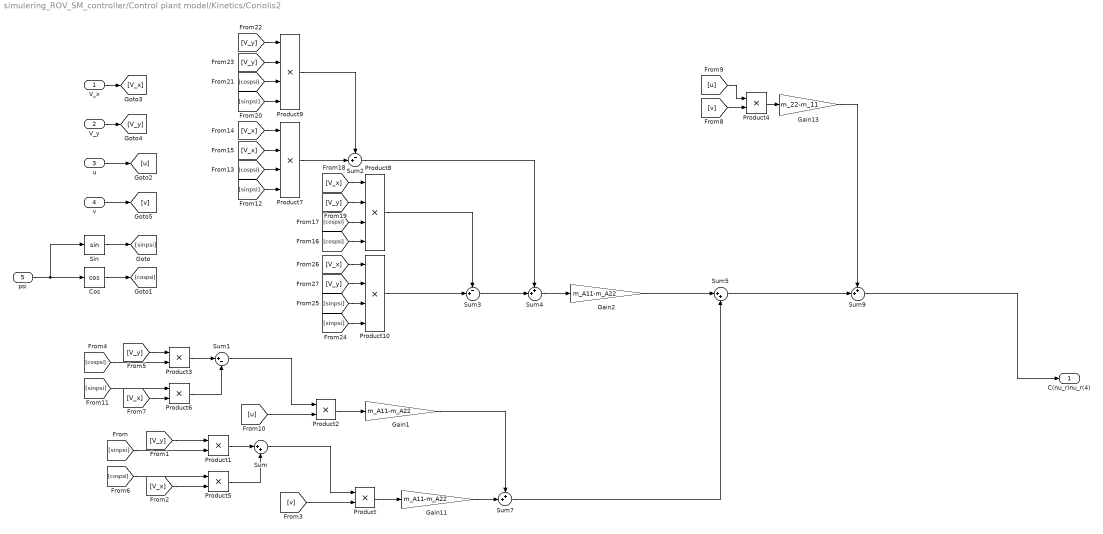
== system simulering_ROV_SM_controller/Control plant model/Kinetics/Coriolis2 ==
  V_x : Inport
  V_y : Inport  Port=2
  u : Inport  Port=3
  v : Inport  Port=4
  psi : Inport  Port=5
  Cos : Trigonometry  Operator=cos
  Gain1 : Gain  Gain=m_A11-m_A22
  Gain11 : Gain  Gain=m_A11-m_A22
  Gain13 : Gain  Gain=m_22-m_11
  Gain2 : Gain  Gain=m_A11-m_A22
  Product{,1..6} (7 alike) : Product
  Product{7..10} (4 alike) : Product  Inputs=4
  Sin : Trigonometry
  Sum : Sum  Inputs=|++
  Sum1 : Sum  Inputs=|+-
  Sum2 : Sum  Inputs=-+|
  Sum3 : Sum  Inputs=-+|
  Sum4 : Sum  Inputs=++|
  Sum5 : Sum  Inputs=|++
  Sum7 : Sum  Inputs=++|
  Sum9 : Sum  Inputs=++|
  C(nu_r)nu_r(4) : Outport
  wires:
  [v] -> Product4/2
  Product4/1 -> Gain13/1
  Product/1 -> Gain11/1
  [v] -> Product/2
  Gain11/1 -> Sum7/2
  [u] -> Product4/1
  Sum9/1 -> C(nu_r)nu_r(4)/1
  psi/1 -> Sin/1, Cos/1
  Sin/1 -> [sinpsi]
  Cos/1 -> [cospsi]
  u/1 -> [u]
  V_x/1 -> [V_x]
  V_y/1 -> [V_y]
  v/1 -> [v]
  Gain13/1 -> Sum9/1
  [V_y] -> Product1/1
  [V_x] -> Product5/2
  Product1/1 -> Sum/1
  Product5/1 -> Sum/2
  Sum/1 -> Product/1
  [sinpsi] -> Product1/2
  [cospsi] -> Product5/1
  Product2/1 -> Gain1/1
  [u] -> Product2/2
  [V_x] -> Product6/2
  Sum1/1 -> Product2/1
  [cospsi] -> Product3/2
  [V_y] -> Product3/1
  [sinpsi] -> Product6/1
  Product3/1 -> Sum1/1
  Product6/1 -> Sum1/2
  Gain1/1 -> Sum7/1
  [sinpsi] -> Product7/4
  [cospsi] -> Product7/3
  [V_x] -> Product7/1
  [V_x] -> Product7/2
  [sinpsi] -> Product9/4
  [V_y] -> Product9/1
  [cospsi] -> Product9/3
  [V_y] -> Product9/2
  Product7/1 -> Sum2/2
  Product9/1 -> Sum2/1
  [V_y] -> Product8/2
  [cospsi] -> Product8/3
  [V_x] -> Product8/1
  Product8/1 -> Sum3/1
  [cospsi] -> Product8/4
  [V_y] -> Product10/2
  [sinpsi] -> Product10/3
  [V_x] -> Product10/1
  [sinpsi] -> Product10/4
  Product10/1 -> Sum3/2
  Sum3/1 -> Sum4/2
  Sum2/1 -> Sum4/1
  Sum4/1 -> Gain2/1
  Sum7/1 -> Sum5/2
  Sum5/1 -> Sum9/2
  Gain2/1 -> Sum5/1

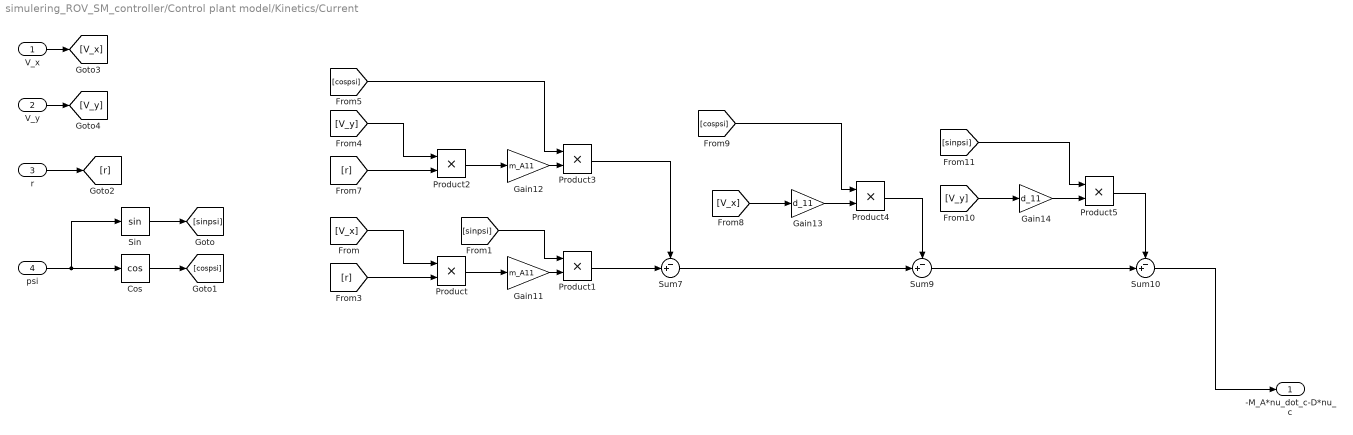
== system simulering_ROV_SM_controller/Control plant model/Kinetics/Current ==
  V_x : Inport
  V_y : Inport  Port=2
  r : Inport  Port=3
  psi : Inport  Port=4
  Cos : Trigonometry  Operator=cos
  Gain11 : Gain  Gain=m_A11
  Gain12 : Gain  Gain=m_A11
  Gain13 : Gain  Gain=d_11
  Gain14 : Gain  Gain=d_11
  Product{,1..5} (6 alike) : Product
  Sin : Trigonometry
  Sum10 : Sum  Inputs=-+|
  Sum7 : Sum  Inputs=-+|
  Sum9 : Sum  Inputs=-+|
  -M_A*nu_dot_c-D*nu_c : Outport
  wires:
  Gain11/1 -> Product1/2
  Product2/1 -> Gain12/1
  [cospsi] -> Product3/1
  [r] -> Product2/2
  Gain13/1 -> Product4/2
  Product4/1 -> Sum9/1
  [V_x] -> Product/1
  Product3/1 -> Sum7/1
  Gain12/1 -> Product3/2
  Product/1 -> Gain11/1
  [V_y] -> Product2/1
  [r] -> Product/2
  Product1/1 -> Sum7/2
  [sinpsi] -> Product1/1
  Gain14/1 -> Product5/2
  [sinpsi] -> Product5/1
  Sum7/1 -> Sum9/2
  [cospsi] -> Product4/1
  [V_y] -> Gain14/1
  [V_x] -> Gain13/1
  Product5/1 -> Sum10/1
  Sum9/1 -> Sum10/2
  Sum10/1 -> -M_A*nu_dot_c-D*nu_c/1
  psi/1 -> Sin/1, Cos/1
  Sin/1 -> [sinpsi]
  Cos/1 -> [cospsi]
  r/1 -> [r]
  V_x/1 -> [V_x]
  V_y/1 -> [V_y]

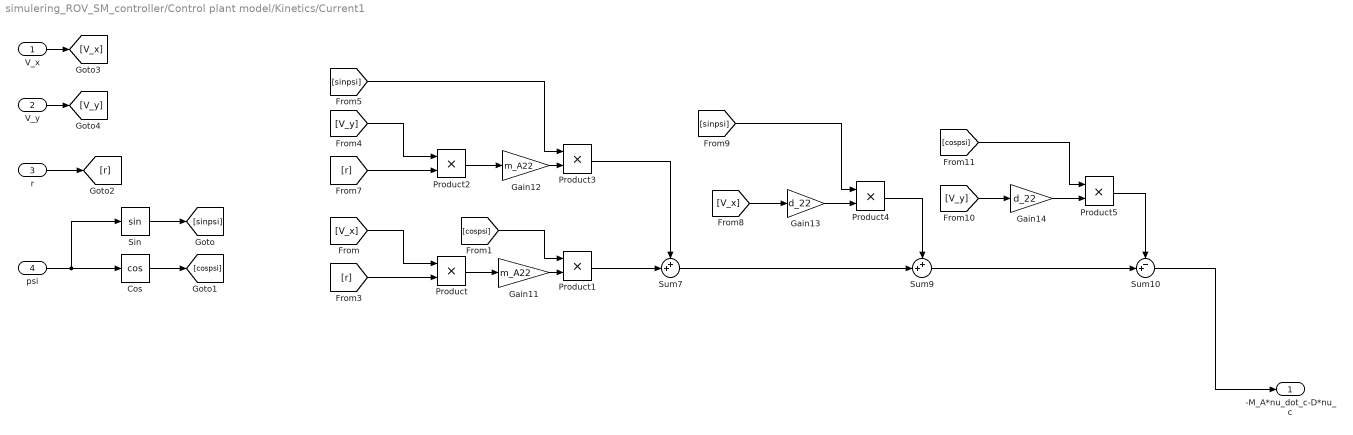
== system simulering_ROV_SM_controller/Control plant model/Kinetics/Current1 ==
  V_x : Inport
  V_y : Inport  Port=2
  r : Inport  Port=3
  psi : Inport  Port=4
  Cos : Trigonometry  Operator=cos
  Gain11 : Gain  Gain=m_A22
  Gain12 : Gain  Gain=m_A22
  Gain13 : Gain  Gain=d_22
  Gain14 : Gain  Gain=d_22
  Product{,1..5} (6 alike) : Product
  Sin : Trigonometry
  Sum10 : Sum  Inputs=-+|
  Sum7 : Sum  Inputs=++|
  Sum9 : Sum  Inputs=++|
  -M_A*nu_dot_c-D*nu_c : Outport
  wires:
  Gain11/1 -> Product1/2
  Product2/1 -> Gain12/1
  [sinpsi] -> Product3/1
  [r] -> Product2/2
  Gain13/1 -> Product4/2
  Product4/1 -> Sum9/1
  [V_x] -> Product/1
  Product3/1 -> Sum7/1
  Gain12/1 -> Product3/2
  Product/1 -> Gain11/1
  [V_y] -> Product2/1
  [r] -> Product/2
  Product1/1 -> Sum7/2
  [cospsi] -> Product1/1
  Gain14/1 -> Product5/2
  [cospsi] -> Product5/1
  Sum7/1 -> Sum9/2
  [sinpsi] -> Product4/1
  [V_y] -> Gain14/1
  [V_x] -> Gain13/1
  Product5/1 -> Sum10/1
  Sum9/1 -> Sum10/2
  Sum10/1 -> -M_A*nu_dot_c-D*nu_c/1
  psi/1 -> Sin/1, Cos/1
  Sin/1 -> [sinpsi]
  Cos/1 -> [cospsi]
  r/1 -> [r]
  V_x/1 -> [V_x]
  V_y/1 -> [V_y]

== matlab function simulering_ROV_SM_controller/Control law/Yaw controller/SSA ==
  data: u input; y output
function y = fcn(u)
%#codegen

y = ssa(u);
